simulink library "mech_airbag_vrlib"  (Simulink 7.1)
libraries: vrlib x7
settings Model: Creator=arnav  LastModifiedBy=batserve

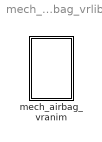
== system mech_airbag_vrlib ==
  mech_airbag_vranim : Subsystem

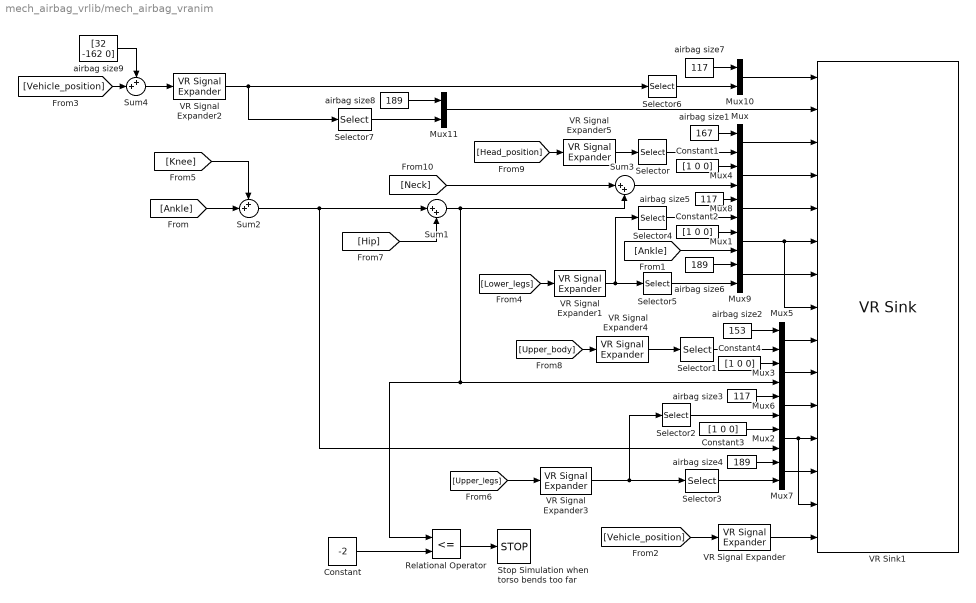
== system mech_airbag_vrlib/mech_airbag_vranim ==
  Constant : Constant  Value=-2  OutDataType=sfix(16)  OutScaling=2^0
  Constant{1..4} (4 alike) : Constant  Value=[1 0 0]  OutDataType=sfix(16)  OutScaling=2^0
  Mux{,1..11} (12 alike) : Mux  Inputs=2
  Relational Operator : RelationalOperator  Operator=<=  ZeroCross=off  InputSameDT=on
  Selector{,1..7} (8 alike) : Selector  InputPortWidth=3  IndexOptions=Index vector (dialog)  Indices=[2 3]  OutputSizes=1
  Stop Simulation when torso bends too far : Stop
  Sum1 : Sum  Inputs=|++  OutDataType=sfix(16)  OutScaling=2^0  SaturateOnIntegerOverflow=on  InputSameDT=on  OutDataTypeStr=Inherit: Same as first input
  Sum2 : Sum  Inputs=++|  OutDataType=sfix(16)  OutScaling=2^0  SaturateOnIntegerOverflow=on  InputSameDT=on  OutDataTypeStr=Inherit: Same as first input
  Sum3 : Sum  Inputs=|++  OutDataType=sfix(16)  OutScaling=2^0  SaturateOnIntegerOverflow=on  InputSameDT=on  OutDataTypeStr=Inherit: Same as first input
  Sum4 : Sum  Inputs=++|  OutDataType=sfix(16)  OutScaling=2^0  SaturateOnIntegerOverflow=on  InputSameDT=on  OutDataTypeStr=Inherit: Same as first input
  VR Signal Expander{,1..5} (6 alike) : vrlib/VR Signal Expander  SystemSampleTime=-1  outwidth=3  outidx=[2 3 1]
  VR Sink1 : vrlib/VR Sink  SampleTime=0.05  ViewEnable=on  RemoteChange=off  RemoteView=off  FieldsWritten=footL.translation#footR.translation#headCOG.translation#headROT.rotation#lowerlegL.translation#lowerlegLROT.rotation#lowerlegR.translation#lowerlegRROT.rotation#torsoCOG.translation#torsoROT.rotation#upperlegL.translation#upperlegLROT.rotation#upperlegR.translation#upperlegRROT.rotation#vehicle.translation  WorldFileName=mech_airbag_world.wrl  WorldDescription=Passenger Collision Model  AutoView=off  VideoDimensions=[]  FigureProperties={}
  airbag size1 : Constant  Value=167  OutDataType=sfix(16)  OutScaling=2^0
  airbag size2 : Constant  Value=153  OutDataType=sfix(16)  OutScaling=2^0
  airbag size3 : Constant  Value=117  OutDataType=sfix(16)  OutScaling=2^0
  airbag size4 : Constant  Value=189  OutDataType=sfix(16)  OutScaling=2^0
  airbag size5 : Constant  Value=117  OutDataType=sfix(16)  OutScaling=2^0
  airbag size6 : Constant  Value=189  OutDataType=sfix(16)  OutScaling=2^0
  airbag size7 : Constant  Value=117  OutDataType=sfix(16)  OutScaling=2^0
  airbag size8 : Constant  Value=189  OutDataType=sfix(16)  OutScaling=2^0
  airbag size9 : Constant  Value=[32 -162 0]  OutDataType=sfix(16)  OutScaling=2^0
  wires:
  Sum3/1 -> Mux4/2
  Mux4/1 -> VR Sink1/4
  Mux3/1 -> VR Sink1/10
  airbag size1/1 -> Mux/1
  Selector/1 -> Mux/2
  Mux/1 -> VR Sink1/3
  Selector1/1 -> Mux5/2
  airbag size3/1 -> Mux6/1
  airbag size4/1 -> Mux7/1
  airbag size6/1 -> Mux9/1
  Selector4/1 -> Mux8/2
  Selector5/1 -> Mux9/2
  Selector7/1 -> Mux11/2
  airbag size8/1 -> Mux11/1
  airbag size7/1 -> Mux10/1
  [Ankle] -> Sum2/2
  [Ankle] -> Mux1/2
  [Vehicle_position] -> VR Signal Expander/1
  [Vehicle_position] -> Sum4/2
  Sum4/1 -> VR Signal Expander2/1
  airbag size9/1 -> Sum4/1
  [Lower_legs] -> VR Signal Expander1/1
  [Hip] -> Sum1/2
  [Upper_body] -> VR Signal Expander4/1
  [Head_position] -> VR Signal Expander5/1
  [Neck] -> Sum3/1
  Selector6/1 -> Mux10/2
  VR Signal Expander2/1 -> Selector7/1, Selector6/1
  VR Signal Expander5/1 -> Selector/1
  Mux10/1 -> VR Sink1/1
  Mux11/1 -> VR Sink1/2
  Constant1/1 -> Mux4/1
  Mux8/1 -> VR Sink1/5
  airbag size5/1 -> Mux8/1
  Mux9/1 -> VR Sink1/7
  Mux1/1 -> VR Sink1/6, VR Sink1/8
  Constant2/1 -> Mux1/1
  Constant4/1 -> Mux3/1
  VR Signal Expander1/1 -> Selector5/1, Selector4/1
  Mux5/1 -> VR Sink1/9
  airbag size2/1 -> Mux5/1
  VR Signal Expander4/1 -> Selector1/1
  Constant3/1 -> Mux2/1
  Mux2/1 -> VR Sink1/12, VR Sink1/14
  [Knee] -> Sum2/1
  Sum1/1 -> Sum3/2, Relational Operator/1, Mux3/2
  Sum2/1 -> Sum1/1, Mux2/2
  Mux6/1 -> VR Sink1/11
  Selector2/1 -> Mux6/2
  Mux7/1 -> VR Sink1/13
  Selector3/1 -> Mux7/2
  VR Signal Expander/1 -> VR Sink1/15
  VR Signal Expander3/1 -> Selector3/1, Selector2/1
  [Upper_legs] -> VR Signal Expander3/1
  Constant/1 -> Relational Operator/2
  Relational Operator/1 -> Stop Simulation when torso bends too far/1
